simulink model "effect_of_controller_on_signal_no_controller"  (R2019a)
settings: Solver=VariableStepAuto  StartTime=0.0  StopTime=25  RelTol=1e-3
libraries: dspsrcs4 x2, simulink x2
settings Model: Creator=raxit  LastModifiedBy=raxit

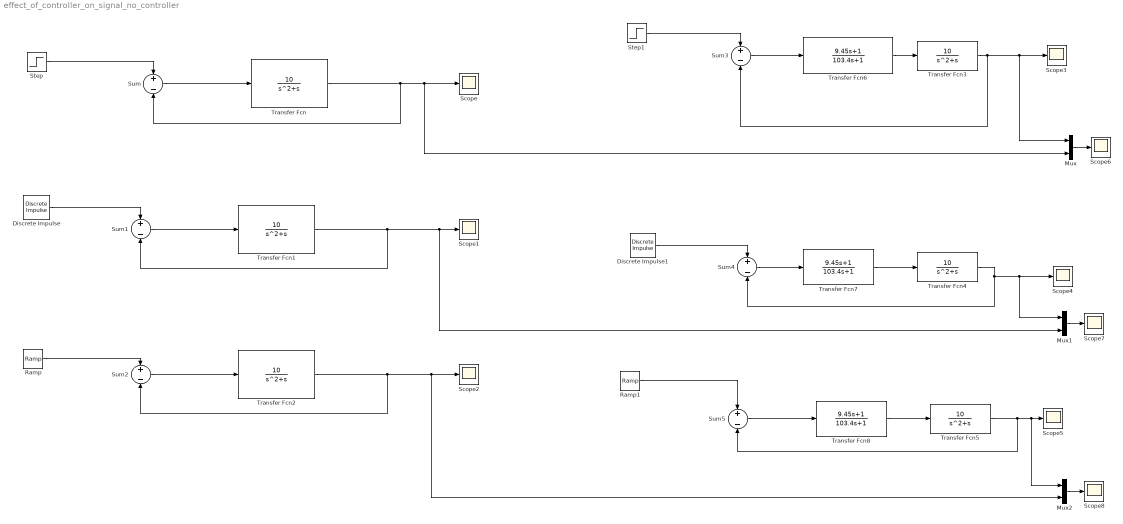
== system effect_of_controller_on_signal_no_controller ==
  Discrete Impulse : dspsrcs4/Discrete  Impulse  Delay=0  SampleTime=1  FrameSample=1  OutputFrames=off  dataType=double  isSigned=on  wordLen=16  udDataType=sfix(16)  fracBitsMode=Best precision  numFracBits=15  OutDataTypeStr=double  LastOutDataTypeStr=double
  Discrete Impulse1 : dspsrcs4/Discrete  Impulse  Delay=0  SampleTime=1  FrameSample=1  OutputFrames=off  dataType=double  isSigned=on  wordLen=16  udDataType=sfix(16)  fracBitsMode=Best precision  numFracBits=15  OutDataTypeStr=double  LastOutDataTypeStr=double
  Mux : Mux  Inputs=2
  Mux1 : Mux  Inputs=2
  Mux2 : Mux  Inputs=2
  Ramp : simulink/Sources/Ramp  slope=1  start=0  InitialOutput=0
  Ramp1 : simulink/Sources/Ramp  slope=1  start=0  InitialOutput=0
  Scope{,1..8} (9 alike) : Scope
  Step : Step  SampleTime=0
  Step1 : Step  SampleTime=0
  Sum{,1..5} (6 alike) : Sum  Inputs=+-
  Transfer Fcn{,1..5} (6 alike) : TransferFcn  Numerator=[10]  Denominator=[1 1 0]
  Transfer Fcn6 : TransferFcn  Numerator=[9.45 1]  Denominator=[103.4 1]
  Transfer Fcn7 : TransferFcn  Numerator=[9.45 1]  Denominator=[103.4 1]
  Transfer Fcn8 : TransferFcn  Numerator=[9.45 1]  Denominator=[103.4 1]
  wires:
  Sum/1 -> Transfer Fcn/1
  Transfer Fcn/1 -> Sum/2, Mux/2, Scope/1
  Step/1 -> Sum/1
  Discrete Impulse/1 -> Sum1/1
  Transfer Fcn1/1 -> Mux1/2, Scope1/1, Sum1/2
  Sum1/1 -> Transfer Fcn1/1
  Ramp/1 -> Sum2/1
  Transfer Fcn2/1 -> Mux2/2, Scope2/1, Sum2/2
  Sum2/1 -> Transfer Fcn2/1
  Discrete Impulse1/1 -> Sum4/1
  Sum3/1 -> Transfer Fcn6/1
  Transfer Fcn6/1 -> Transfer Fcn3/1
  Transfer Fcn5/1 -> Mux2/1, Scope5/1, Sum5/2
  Sum4/1 -> Transfer Fcn7/1
  Transfer Fcn4/1 -> Mux1/1, Scope4/1, Sum4/2
  Transfer Fcn8/1 -> Transfer Fcn5/1
  Transfer Fcn3/1 -> Mux/1, Scope3/1, Sum3/2
  Transfer Fcn7/1 -> Transfer Fcn4/1
  Ramp1/1 -> Sum5/1
  Sum5/1 -> Transfer Fcn8/1
  Step1/1 -> Sum3/1
  Mux/1 -> Scope6/1
  Mux1/1 -> Scope7/1
  Mux2/1 -> Scope8/1
